simulink model "heat_exchanger_test02_sim"  (R2017b)
settings: Solver=VariableStepAuto  StartTime=0.0  StopTime=0  RelTol=1e-3
values from neighbouring files (symbols this model uses):
  c = conversion_factors()    [heat_exchanger_test01.m]    (also in reactor_test_ideal_gas_models_comparison.m)
undefined symbols (not defined in the file or in its folder): CoolProp
libraries: thermochemical x6
settings Model: Creator=fferrucc  LastModifiedBy=fferrucc

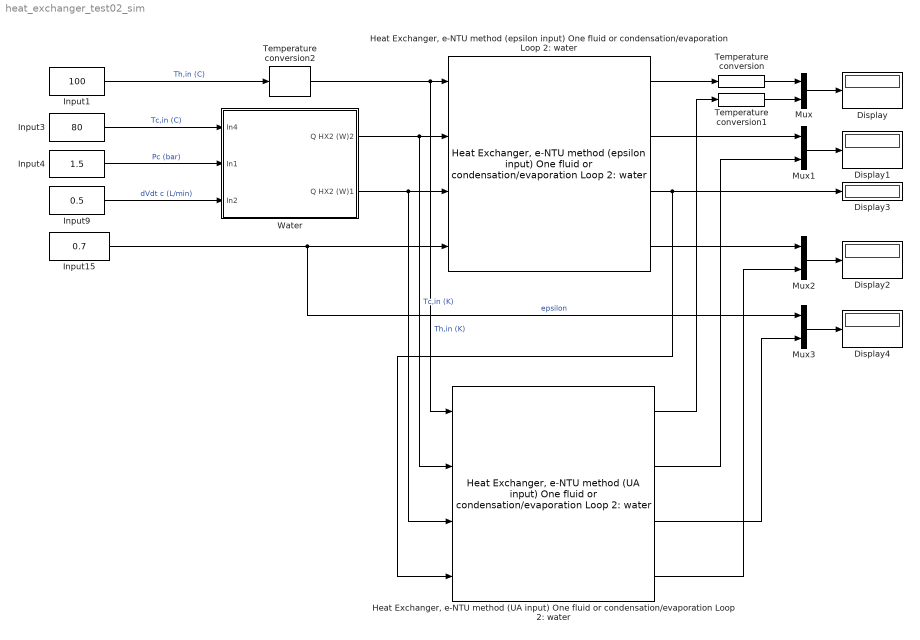
== system heat_exchanger_test02_sim ==
  Display{,1..4} (5 alike) : Display
  "Heat Exchanger, e-NTU method (UA input) One fluid or condensation/evaporation Loop 2: water" : thermochemical/Heat exchangers/Heat Exchanger, e-NTU method (UA input) One fluid or condensation//evaporation Loop 2: water  cp_water_J_K_mol=75.3260
      settings: SourceProductName=@ Thermochemical
  "Heat Exchanger, e-NTU method (epsilon input) One fluid or condensation/evaporation Loop 2: water" : thermochemical/Heat exchangers/Heat Exchanger, e-NTU method (epsilon input) One fluid or condensation//evaporation Loop 2: water  cp_water_J_K_mol=75.3260
      settings: SourceProductName=@ Thermochemical
  Input1 : Constant  Value=100
  Input15 : Constant  Value=0.7
  Input3 : Constant  Value=80
  Input4 : Constant  Value=1.5
  Input9 : Constant  Value=0.5
  Mux{,1..3} (4 alike) : Mux  Inputs=2
  Temperature conversion : thermochemical/Conversions/Temperature conversion  sel=K --> °C
      settings: SourceProductName=@ Thermochemical
  Temperature conversion1 : thermochemical/Conversions/Temperature conversion  sel=K --> °C
      settings: SourceProductName=@ Thermochemical
  Temperature conversion2 : thermochemical/Conversions/Temperature conversion  sel=°C --> K
      settings: SourceProductName=@ Thermochemical
  Water : Subsystem
  wires:
  Input3/1 -> Water/1(In4)  "Tc,in (C)"
  Input4/1 -> Water/2(In1)  "Pc (bar)"
  Input9/1 -> Water/3(In2)  "dVdt c (L/min)"
  Input15/1 -> Mux3/1, "Heat Exchanger, e-NTU method (epsilon input) One fluid or condensation/evaporation Loop 2: water"/4  "epsilon"
  Water/2(Q HX2 (W)1) -> "Heat Exchanger, e-NTU method (UA input) One fluid or condensation/evaporation Loop 2: water"/3, "Heat Exchanger, e-NTU method (epsilon input) One fluid or condensation/evaporation Loop 2: water"/3
  Water/1(Q HX2 (W)2) -> "Heat Exchanger, e-NTU method (UA input) One fluid or condensation/evaporation Loop 2: water"/2, "Heat Exchanger, e-NTU method (epsilon input) One fluid or condensation/evaporation Loop 2: water"/2  "Tc,in (K)"
  Temperature conversion2/1 -> "Heat Exchanger, e-NTU method (UA input) One fluid or condensation/evaporation Loop 2: water"/1, "Heat Exchanger, e-NTU method (epsilon input) One fluid or condensation/evaporation Loop 2: water"/1  "Th,in (K)"
  Mux/1 -> Display/1
  Temperature conversion/1 -> Mux/1
  Temperature conversion1/1 -> Mux/2
  Input1/1 -> Temperature conversion2/1  "Th,in (C)"
  "Heat Exchanger, e-NTU method (epsilon input) One fluid or condensation/evaporation Loop 2: water"/1 -> Temperature conversion/1
  Mux1/1 -> Display1/1
  "Heat Exchanger, e-NTU method (epsilon input) One fluid or condensation/evaporation Loop 2: water"/2 -> Mux1/1
  Mux2/1 -> Display2/1
  "Heat Exchanger, e-NTU method (epsilon input) One fluid or condensation/evaporation Loop 2: water"/4 -> Mux2/1
  "Heat Exchanger, e-NTU method (epsilon input) One fluid or condensation/evaporation Loop 2: water"/3 -> "Heat Exchanger, e-NTU method (UA input) One fluid or condensation/evaporation Loop 2: water"/4, Display3/1
  Mux3/1 -> Display4/1
  "Heat Exchanger, e-NTU method (UA input) One fluid or condensation/evaporation Loop 2: water"/1 -> Temperature conversion1/1
  "Heat Exchanger, e-NTU method (UA input) One fluid or condensation/evaporation Loop 2: water"/2 -> Mux1/2
  "Heat Exchanger, e-NTU method (UA input) One fluid or condensation/evaporation Loop 2: water"/3 -> Mux3/2
  "Heat Exchanger, e-NTU method (UA input) One fluid or condensation/evaporation Loop 2: water"/4 -> Mux2/2

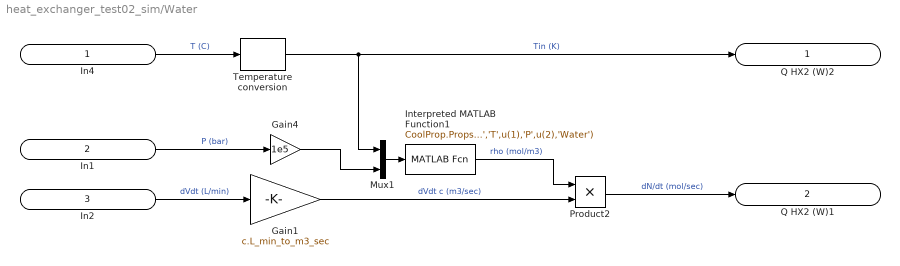
== system heat_exchanger_test02_sim/Water ==
  In4 : Inport
  In1 : Inport  Port=2
  In2 : Inport  Port=3
  Gain1 : Gain  Gain=c.L_min_to_m3_sec
  Gain4 : Gain  Gain=1e5
  Interpreted MATLAB Function1 : MATLABFcn  MATLABFcn=CoolProp.PropsSI('DMOLAR','T',u(1),'P',u(2),'Water')  OutputDimensions=1
  Mux1 : Mux  Inputs=2
  Product2 : Product
  Temperature conversion : thermochemical/Conversions/Temperature conversion  sel=°C --> K
      settings: SourceProductName=@ Thermochemical
  Q HX2 (W)2 : Outport
  Q HX2 (W)1 : Outport  Port=2
  wires:
  Mux1/1 -> Interpreted MATLAB Function1/1
  Interpreted MATLAB Function1/1 -> Product2/1  "rho (mol/m3)"
  Temperature conversion/1 -> Q HX2 (W)2/1, Mux1/1  "Tin (K)"
  Gain4/1 -> Mux1/2
  Product2/1 -> Q HX2 (W)1/1  "dN/dt (mol/sec)"
  In2/1 -> Gain1/1  "dVdt (L/min)"
  In4/1 -> Temperature conversion/1  "T (C)"
  Gain1/1 -> Product2/2  "dVdt c (m3/sec)"
  In1/1 -> Gain4/1  "P (bar)"
